simulink model "tx2"  (R2022a)
settings: Solver=FixedStepDiscrete  StartTime=0.0  StopTime=3.1e6  FixedStep=1  RelTol=1e-3
undefined symbols (not defined in the file or in its folder): rom_bf1, rom_bf2, rom_bf3, rom_bf4, rom_bf5, rom_bf6, rom_bf7, rom_bf8, rom_pilot_tt
libraries: hdlsllib x809, whdlutilities x460, whdlmod x104, whdledac x26, simulink x3
(part 20 of 27)

== system tx2/Subsystem7/OFDM_process1/OFDM_process1_bf1/OFDM_BF1 ==
  data : Inport  OutDataTypeStr=fixdt(1,16,14)  LockScale=on
      settings: SignalType=complex
  OFDM_ctrl : Inport  Port=2  OutDataTypeStr=Bus: samplecontrol
  Constant : Constant  Value=0  OutDataTypeStr=boolean
  Data Type Conversion : DataTypeConversion  OutDataTypeStr=boolean  SaturateOnIntegerOverflow=off  RndMeth=Floor
  Delay : Delay  DelayLength=1  InitialCondition=0
  HDL Counter : hdlsllib/Sources/HDL Counter  CountType=Count limited  CountInit=0  CountStep=1  CountMax=1  CountFromType=Initial value  CountFrom=0  CountResetPort=on  CountLoadPort=off  CountEnbPort=on  CountDirPort=off  CountHitOutputPort=off  CountDataType=Unsigned  CountWordLen=8  CountFracLen=0  CountSampTime=1
  HDL Counter1 : hdlsllib/Sources/HDL Counter  CountType=Count limited  CountInit=1  CountStep=1  CountMax=232+cp-1  CountFromType=Initial value  CountFrom=1  CountResetPort=on  CountLoadPort=off  CountEnbPort=on  CountDirPort=off  CountHitOutputPort=on  CountDataType=Unsigned  CountWordLen=10  CountFracLen=0  CountSampTime=1
  Logical Operator1 : Logic  Operator=NOT  AllPortsSameDT=off  OutDataTypeStr=boolean
  OFDM Modulator long prefix : whdlmod/OFDM Modulator  OFDMParametersSource=Property  FFTLength=1024  MaxFFTLength=64  CPLength=cp  numLgSc=0  numRgSc=0  InsertDCNull=off  Windowing=off  WindowLength=cp  MaxWindowLength=8  ResetInputPort=on  Normalize=on  RoundingMethod=Floor  SimulateUsing=Code generation
      settings: SourceProductBaseCode=LH
  Sample Control Bus Selector : whdlutilities/Sample Control Bus Selector  OutputSignals=start,end,valid
      settings: SourceProductBaseCode=LH
  recover_valid_specify : Subsystem  AncestorBlock=mylib/rate_match_L2/interleave/recover_valid_specify
  data_out : Outport  VectorParamsAs1DForOutWhenUnconnected=off
  valid_out : Outport  Port=2  VectorParamsAs1DForOutWhenUnconnected=off
  wires:
  OFDM Modulator long prefix/1 -> data_out/1
  data/1 -> recover_valid_specify/1(data_in)
  OFDM Modulator long prefix/2 -> valid_out/1
  OFDM_ctrl/1 -> Sample Control Bus Selector/1
  Sample Control Bus Selector/2 -> HDL Counter/2  "<end>"
  HDL Counter/1 -> Data Type Conversion/1
  Data Type Conversion/1 -> Logical Operator1/1, HDL Counter1/2
  HDL Counter1/2 -> Delay/1, HDL Counter/1
  Logical Operator1/1 -> HDL Counter1/1
  Sample Control Bus Selector/1 -> recover_valid_specify/2(start_in)  "<start>"
  Delay/1 -> recover_valid_specify/3(end_in)
  recover_valid_specify/1(data_out) -> OFDM Modulator long prefix/1
  recover_valid_specify/4(valid_out) -> OFDM Modulator long prefix/2
  Constant/1 -> OFDM Modulator long prefix/3

== system tx2/Subsystem7/OFDM_process1/OFDM_process1_bf1/ctrl_gen ==
  data_in : Inport
      settings: SignalType=complex
  valid_in : Inport  Port=2
  Delay : Delay  DelayLength=1  InitialCondition=0
  Delay1 : Delay  DelayLength=1  InitialCondition=0
  Delay2 : Delay  DelayLength=1  InitialCondition=0
  Detect Fall Nonpositive : hdlsllib/Logic and Bit Operations/Detect Fall Nonpositive  vinit=0  OutDataTypeStr=boolean
      settings: SourceProductBaseCode=SL
  Detect Rise Positive : hdlsllib/Logic and Bit Operations/Detect Rise Positive  vinit=0  OutDataTypeStr=boolean
      settings: SourceProductBaseCode=SL
  Sample Control Bus Creator : whdlutilities/Sample Control Bus Creator
      settings: SourceProductBaseCode=LH
  data_out : Outport
  ctrl_out : Outport  Port=2
  wires:
  Delay2/1 -> data_out/1
  data_in/1 -> Delay2/1
  Delay1/1 -> Detect Rise Positive/1
  Delay/1 -> Sample Control Bus Creator/3
  Sample Control Bus Creator/1 -> ctrl_out/1
  valid_in/1 -> Delay1/1, Detect Fall Nonpositive/1, Delay/1
  Detect Rise Positive/1 -> Sample Control Bus Creator/1
  Detect Fall Nonpositive/1 -> Sample Control Bus Creator/2

== system tx2/Subsystem7/OFDM_process1/OFDM_process1_bf2/OFDM_BF1 ==
  data : Inport  OutDataTypeStr=fixdt(1,16,14)  LockScale=on
      settings: SignalType=complex
  OFDM_ctrl : Inport  Port=2  OutDataTypeStr=Bus: samplecontrol
  Constant : Constant  Value=0  OutDataTypeStr=boolean
  Data Type Conversion : DataTypeConversion  OutDataTypeStr=boolean  SaturateOnIntegerOverflow=off  RndMeth=Floor
  Delay : Delay  DelayLength=1  InitialCondition=0
  HDL Counter : hdlsllib/Sources/HDL Counter  CountType=Count limited  CountInit=0  CountStep=1  CountMax=1  CountFromType=Initial value  CountFrom=0  CountResetPort=on  CountLoadPort=off  CountEnbPort=on  CountDirPort=off  CountHitOutputPort=off  CountDataType=Unsigned  CountWordLen=8  CountFracLen=0  CountSampTime=1
  HDL Counter1 : hdlsllib/Sources/HDL Counter  CountType=Count limited  CountInit=1  CountStep=1  CountMax=232+cp-1  CountFromType=Initial value  CountFrom=1  CountResetPort=on  CountLoadPort=off  CountEnbPort=on  CountDirPort=off  CountHitOutputPort=on  CountDataType=Unsigned  CountWordLen=10  CountFracLen=0  CountSampTime=1
  Logical Operator1 : Logic  Operator=NOT  AllPortsSameDT=off  OutDataTypeStr=boolean
  OFDM Modulator long prefix : whdlmod/OFDM Modulator  OFDMParametersSource=Property  FFTLength=1024  MaxFFTLength=64  CPLength=cp  numLgSc=0  numRgSc=0  InsertDCNull=off  Windowing=off  WindowLength=cp  MaxWindowLength=8  ResetInputPort=on  Normalize=on  RoundingMethod=Floor  SimulateUsing=Code generation
      settings: SourceProductBaseCode=LH
  Sample Control Bus Selector : whdlutilities/Sample Control Bus Selector  OutputSignals=start,end,valid
      settings: SourceProductBaseCode=LH
  recover_valid_specify : Subsystem  AncestorBlock=mylib/rate_match_L2/interleave/recover_valid_specify
  data_out : Outport  VectorParamsAs1DForOutWhenUnconnected=off
  valid_out : Outport  Port=2  VectorParamsAs1DForOutWhenUnconnected=off
  wires:
  Constant/1 -> OFDM Modulator long prefix/3
  recover_valid_specify/4(valid_out) -> OFDM Modulator long prefix/2
  recover_valid_specify/1(data_out) -> OFDM Modulator long prefix/1
  Delay/1 -> recover_valid_specify/3(end_in)
  Sample Control Bus Selector/1 -> recover_valid_specify/2(start_in)  "<start>"
  Logical Operator1/1 -> HDL Counter1/1
  HDL Counter1/2 -> HDL Counter/1, Delay/1
  Data Type Conversion/1 -> HDL Counter1/2, Logical Operator1/1
  HDL Counter/1 -> Data Type Conversion/1
  Sample Control Bus Selector/2 -> HDL Counter/2  "<end>"
  OFDM_ctrl/1 -> Sample Control Bus Selector/1
  OFDM Modulator long prefix/2 -> valid_out/1
  data/1 -> recover_valid_specify/1(data_in)
  OFDM Modulator long prefix/1 -> data_out/1

== system tx2/Subsystem7/OFDM_process1/OFDM_process1_bf2/ctrl_gen ==
  data_in : Inport
      settings: SignalType=complex
  valid_in : Inport  Port=2
  Delay : Delay  DelayLength=1  InitialCondition=0
  Delay1 : Delay  DelayLength=1  InitialCondition=0
  Delay2 : Delay  DelayLength=1  InitialCondition=0
  Detect Fall Nonpositive : hdlsllib/Logic and Bit Operations/Detect Fall Nonpositive  vinit=0  OutDataTypeStr=boolean
      settings: SourceProductBaseCode=SL
  Detect Rise Positive : hdlsllib/Logic and Bit Operations/Detect Rise Positive  vinit=0  OutDataTypeStr=boolean
      settings: SourceProductBaseCode=SL
  Sample Control Bus Creator : whdlutilities/Sample Control Bus Creator
      settings: SourceProductBaseCode=LH
  data_out : Outport
  ctrl_out : Outport  Port=2
  wires:
  Detect Fall Nonpositive/1 -> Sample Control Bus Creator/2
  Detect Rise Positive/1 -> Sample Control Bus Creator/1
  valid_in/1 -> Delay/1, Detect Fall Nonpositive/1, Delay1/1
  Sample Control Bus Creator/1 -> ctrl_out/1
  Delay/1 -> Sample Control Bus Creator/3
  Delay1/1 -> Detect Rise Positive/1
  data_in/1 -> Delay2/1
  Delay2/1 -> data_out/1

== system tx2/Subsystem7/OFDM_process1/OFDM_process1_bf3/OFDM_BF1 ==
  data : Inport  OutDataTypeStr=fixdt(1,16,14)  LockScale=on
      settings: SignalType=complex
  OFDM_ctrl : Inport  Port=2  OutDataTypeStr=Bus: samplecontrol
  Constant : Constant  Value=0  OutDataTypeStr=boolean
  Data Type Conversion : DataTypeConversion  OutDataTypeStr=boolean  SaturateOnIntegerOverflow=off  RndMeth=Floor
  Delay : Delay  DelayLength=1  InitialCondition=0
  HDL Counter : hdlsllib/Sources/HDL Counter  CountType=Count limited  CountInit=0  CountStep=1  CountMax=1  CountFromType=Initial value  CountFrom=0  CountResetPort=on  CountLoadPort=off  CountEnbPort=on  CountDirPort=off  CountHitOutputPort=off  CountDataType=Unsigned  CountWordLen=8  CountFracLen=0  CountSampTime=1
  HDL Counter1 : hdlsllib/Sources/HDL Counter  CountType=Count limited  CountInit=1  CountStep=1  CountMax=232+cp-1  CountFromType=Initial value  CountFrom=1  CountResetPort=on  CountLoadPort=off  CountEnbPort=on  CountDirPort=off  CountHitOutputPort=on  CountDataType=Unsigned  CountWordLen=10  CountFracLen=0  CountSampTime=1
  Logical Operator1 : Logic  Operator=NOT  AllPortsSameDT=off  OutDataTypeStr=boolean
  OFDM Modulator long prefix : whdlmod/OFDM Modulator  OFDMParametersSource=Property  FFTLength=1024  MaxFFTLength=64  CPLength=cp  numLgSc=0  numRgSc=0  InsertDCNull=off  Windowing=off  WindowLength=cp  MaxWindowLength=8  ResetInputPort=on  Normalize=on  RoundingMethod=Floor  SimulateUsing=Code generation
      settings: SourceProductBaseCode=LH
  Sample Control Bus Selector : whdlutilities/Sample Control Bus Selector  OutputSignals=start,end,valid
      settings: SourceProductBaseCode=LH
  recover_valid_specify : Subsystem  AncestorBlock=mylib/rate_match_L2/interleave/recover_valid_specify
  data_out : Outport  VectorParamsAs1DForOutWhenUnconnected=off
  valid_out : Outport  Port=2  VectorParamsAs1DForOutWhenUnconnected=off
  wires:
  OFDM Modulator long prefix/1 -> data_out/1
  data/1 -> recover_valid_specify/1(data_in)
  OFDM Modulator long prefix/2 -> valid_out/1
  OFDM_ctrl/1 -> Sample Control Bus Selector/1
  Sample Control Bus Selector/2 -> HDL Counter/2  "<end>"
  HDL Counter/1 -> Data Type Conversion/1
  Data Type Conversion/1 -> Logical Operator1/1, HDL Counter1/2
  HDL Counter1/2 -> Delay/1, HDL Counter/1
  Logical Operator1/1 -> HDL Counter1/1
  Sample Control Bus Selector/1 -> recover_valid_specify/2(start_in)  "<start>"
  Delay/1 -> recover_valid_specify/3(end_in)
  recover_valid_specify/1(data_out) -> OFDM Modulator long prefix/1
  recover_valid_specify/4(valid_out) -> OFDM Modulator long prefix/2
  Constant/1 -> OFDM Modulator long prefix/3

== system tx2/Subsystem7/OFDM_process1/OFDM_process1_bf3/ctrl_gen ==
  data_in : Inport
      settings: SignalType=complex
  valid_in : Inport  Port=2
  Delay : Delay  DelayLength=1  InitialCondition=0
  Delay1 : Delay  DelayLength=1  InitialCondition=0
  Delay2 : Delay  DelayLength=1  InitialCondition=0
  Detect Fall Nonpositive : hdlsllib/Logic and Bit Operations/Detect Fall Nonpositive  vinit=0  OutDataTypeStr=boolean
      settings: SourceProductBaseCode=SL
  Detect Rise Positive : hdlsllib/Logic and Bit Operations/Detect Rise Positive  vinit=0  OutDataTypeStr=boolean
      settings: SourceProductBaseCode=SL
  Sample Control Bus Creator : whdlutilities/Sample Control Bus Creator
      settings: SourceProductBaseCode=LH
  data_out : Outport
  ctrl_out : Outport  Port=2
  wires:
  Delay2/1 -> data_out/1
  data_in/1 -> Delay2/1
  Delay1/1 -> Detect Rise Positive/1
  Delay/1 -> Sample Control Bus Creator/3
  Sample Control Bus Creator/1 -> ctrl_out/1
  valid_in/1 -> Delay1/1, Detect Fall Nonpositive/1, Delay/1
  Detect Rise Positive/1 -> Sample Control Bus Creator/1
  Detect Fall Nonpositive/1 -> Sample Control Bus Creator/2

== system tx2/Subsystem7/OFDM_process1/OFDM_process1_bf4/OFDM_BF1 ==
  data : Inport  OutDataTypeStr=fixdt(1,16,14)  LockScale=on
      settings: SignalType=complex
  OFDM_ctrl : Inport  Port=2  OutDataTypeStr=Bus: samplecontrol
  Constant : Constant  Value=0  OutDataTypeStr=boolean
  Data Type Conversion : DataTypeConversion  OutDataTypeStr=boolean  SaturateOnIntegerOverflow=off  RndMeth=Floor
  Delay : Delay  DelayLength=1  InitialCondition=0
  HDL Counter : hdlsllib/Sources/HDL Counter  CountType=Count limited  CountInit=0  CountStep=1  CountMax=1  CountFromType=Initial value  CountFrom=0  CountResetPort=on  CountLoadPort=off  CountEnbPort=on  CountDirPort=off  CountHitOutputPort=off  CountDataType=Unsigned  CountWordLen=8  CountFracLen=0  CountSampTime=1
  HDL Counter1 : hdlsllib/Sources/HDL Counter  CountType=Count limited  CountInit=1  CountStep=1  CountMax=232+cp-1  CountFromType=Initial value  CountFrom=1  CountResetPort=on  CountLoadPort=off  CountEnbPort=on  CountDirPort=off  CountHitOutputPort=on  CountDataType=Unsigned  CountWordLen=10  CountFracLen=0  CountSampTime=1
  Logical Operator1 : Logic  Operator=NOT  AllPortsSameDT=off  OutDataTypeStr=boolean
  OFDM Modulator long prefix : whdlmod/OFDM Modulator  OFDMParametersSource=Property  FFTLength=1024  MaxFFTLength=64  CPLength=cp  numLgSc=0  numRgSc=0  InsertDCNull=off  Windowing=off  WindowLength=cp  MaxWindowLength=8  ResetInputPort=on  Normalize=on  RoundingMethod=Floor  SimulateUsing=Code generation
      settings: SourceProductBaseCode=LH
  Sample Control Bus Selector : whdlutilities/Sample Control Bus Selector  OutputSignals=start,end,valid
      settings: SourceProductBaseCode=LH
  recover_valid_specify : Subsystem  AncestorBlock=mylib/rate_match_L2/interleave/recover_valid_specify
  data_out : Outport  VectorParamsAs1DForOutWhenUnconnected=off
  valid_out : Outport  Port=2  VectorParamsAs1DForOutWhenUnconnected=off
  wires:
  Constant/1 -> OFDM Modulator long prefix/3
  recover_valid_specify/4(valid_out) -> OFDM Modulator long prefix/2
  recover_valid_specify/1(data_out) -> OFDM Modulator long prefix/1
  Delay/1 -> recover_valid_specify/3(end_in)
  Sample Control Bus Selector/1 -> recover_valid_specify/2(start_in)  "<start>"
  Logical Operator1/1 -> HDL Counter1/1
  HDL Counter1/2 -> HDL Counter/1, Delay/1
  Data Type Conversion/1 -> HDL Counter1/2, Logical Operator1/1
  HDL Counter/1 -> Data Type Conversion/1
  Sample Control Bus Selector/2 -> HDL Counter/2  "<end>"
  OFDM_ctrl/1 -> Sample Control Bus Selector/1
  OFDM Modulator long prefix/2 -> valid_out/1
  data/1 -> recover_valid_specify/1(data_in)
  OFDM Modulator long prefix/1 -> data_out/1

== system tx2/Subsystem7/OFDM_process1/OFDM_process1_bf4/ctrl_gen ==
  data_in : Inport
      settings: SignalType=complex
  valid_in : Inport  Port=2
  Delay : Delay  DelayLength=1  InitialCondition=0
  Delay1 : Delay  DelayLength=1  InitialCondition=0
  Delay2 : Delay  DelayLength=1  InitialCondition=0
  Detect Fall Nonpositive : hdlsllib/Logic and Bit Operations/Detect Fall Nonpositive  vinit=0  OutDataTypeStr=boolean
      settings: SourceProductBaseCode=SL
  Detect Rise Positive : hdlsllib/Logic and Bit Operations/Detect Rise Positive  vinit=0  OutDataTypeStr=boolean
      settings: SourceProductBaseCode=SL
  Sample Control Bus Creator : whdlutilities/Sample Control Bus Creator
      settings: SourceProductBaseCode=LH
  data_out : Outport
  ctrl_out : Outport  Port=2
  wires:
  Detect Fall Nonpositive/1 -> Sample Control Bus Creator/2
  Detect Rise Positive/1 -> Sample Control Bus Creator/1
  valid_in/1 -> Delay/1, Detect Fall Nonpositive/1, Delay1/1
  Sample Control Bus Creator/1 -> ctrl_out/1
  Delay/1 -> Sample Control Bus Creator/3
  Delay1/1 -> Detect Rise Positive/1
  data_in/1 -> Delay2/1
  Delay2/1 -> data_out/1

== system tx2/Subsystem7/OFDM_process1/OFDM_process1_bf5/OFDM_BF1 ==
  data : Inport  OutDataTypeStr=fixdt(1,16,14)  LockScale=on
      settings: SignalType=complex
  OFDM_ctrl : Inport  Port=2  OutDataTypeStr=Bus: samplecontrol
  Constant : Constant  Value=0  OutDataTypeStr=boolean
  Data Type Conversion : DataTypeConversion  OutDataTypeStr=boolean  SaturateOnIntegerOverflow=off  RndMeth=Floor
  Delay : Delay  DelayLength=1  InitialCondition=0
  HDL Counter : hdlsllib/Sources/HDL Counter  CountType=Count limited  CountInit=0  CountStep=1  CountMax=1  CountFromType=Initial value  CountFrom=0  CountResetPort=on  CountLoadPort=off  CountEnbPort=on  CountDirPort=off  CountHitOutputPort=off  CountDataType=Unsigned  CountWordLen=8  CountFracLen=0  CountSampTime=1
  HDL Counter1 : hdlsllib/Sources/HDL Counter  CountType=Count limited  CountInit=1  CountStep=1  CountMax=232+cp-1  CountFromType=Initial value  CountFrom=1  CountResetPort=on  CountLoadPort=off  CountEnbPort=on  CountDirPort=off  CountHitOutputPort=on  CountDataType=Unsigned  CountWordLen=10  CountFracLen=0  CountSampTime=1
  Logical Operator1 : Logic  Operator=NOT  AllPortsSameDT=off  OutDataTypeStr=boolean
  OFDM Modulator long prefix : whdlmod/OFDM Modulator  OFDMParametersSource=Property  FFTLength=1024  MaxFFTLength=64  CPLength=cp  numLgSc=0  numRgSc=0  InsertDCNull=off  Windowing=off  WindowLength=cp  MaxWindowLength=8  ResetInputPort=on  Normalize=on  RoundingMethod=Floor  SimulateUsing=Code generation
      settings: SourceProductBaseCode=LH
  Sample Control Bus Selector : whdlutilities/Sample Control Bus Selector  OutputSignals=start,end,valid
      settings: SourceProductBaseCode=LH
  recover_valid_specify : Subsystem  AncestorBlock=mylib/rate_match_L2/interleave/recover_valid_specify
  data_out : Outport  VectorParamsAs1DForOutWhenUnconnected=off
  valid_out : Outport  Port=2  VectorParamsAs1DForOutWhenUnconnected=off
  wires:
  OFDM Modulator long prefix/1 -> data_out/1
  data/1 -> recover_valid_specify/1(data_in)
  OFDM Modulator long prefix/2 -> valid_out/1
  OFDM_ctrl/1 -> Sample Control Bus Selector/1
  Sample Control Bus Selector/2 -> HDL Counter/2  "<end>"
  HDL Counter/1 -> Data Type Conversion/1
  Data Type Conversion/1 -> Logical Operator1/1, HDL Counter1/2
  HDL Counter1/2 -> Delay/1, HDL Counter/1
  Logical Operator1/1 -> HDL Counter1/1
  Sample Control Bus Selector/1 -> recover_valid_specify/2(start_in)  "<start>"
  Delay/1 -> recover_valid_specify/3(end_in)
  recover_valid_specify/1(data_out) -> OFDM Modulator long prefix/1
  recover_valid_specify/4(valid_out) -> OFDM Modulator long prefix/2
  Constant/1 -> OFDM Modulator long prefix/3

== system tx2/Subsystem7/OFDM_process1/OFDM_process1_bf5/ctrl_gen ==
  data_in : Inport
      settings: SignalType=complex
  valid_in : Inport  Port=2
  Delay : Delay  DelayLength=1  InitialCondition=0
  Delay1 : Delay  DelayLength=1  InitialCondition=0
  Delay2 : Delay  DelayLength=1  InitialCondition=0
  Detect Fall Nonpositive : hdlsllib/Logic and Bit Operations/Detect Fall Nonpositive  vinit=0  OutDataTypeStr=boolean
      settings: SourceProductBaseCode=SL
  Detect Rise Positive : hdlsllib/Logic and Bit Operations/Detect Rise Positive  vinit=0  OutDataTypeStr=boolean
      settings: SourceProductBaseCode=SL
  Sample Control Bus Creator : whdlutilities/Sample Control Bus Creator
      settings: SourceProductBaseCode=LH
  data_out : Outport
  ctrl_out : Outport  Port=2
  wires:
  Delay2/1 -> data_out/1
  data_in/1 -> Delay2/1
  Delay1/1 -> Detect Rise Positive/1
  Delay/1 -> Sample Control Bus Creator/3
  Sample Control Bus Creator/1 -> ctrl_out/1
  valid_in/1 -> Delay1/1, Detect Fall Nonpositive/1, Delay/1
  Detect Rise Positive/1 -> Sample Control Bus Creator/1
  Detect Fall Nonpositive/1 -> Sample Control Bus Creator/2

== system tx2/Subsystem7/OFDM_process1/OFDM_process1_bf6/OFDM_BF1 ==
  data : Inport  OutDataTypeStr=fixdt(1,16,14)  LockScale=on
      settings: SignalType=complex
  OFDM_ctrl : Inport  Port=2  OutDataTypeStr=Bus: samplecontrol
  Constant : Constant  Value=0  OutDataTypeStr=boolean
  Data Type Conversion : DataTypeConversion  OutDataTypeStr=boolean  SaturateOnIntegerOverflow=off  RndMeth=Floor
  Delay : Delay  DelayLength=1  InitialCondition=0
  HDL Counter : hdlsllib/Sources/HDL Counter  CountType=Count limited  CountInit=0  CountStep=1  CountMax=1  CountFromType=Initial value  CountFrom=0  CountResetPort=on  CountLoadPort=off  CountEnbPort=on  CountDirPort=off  CountHitOutputPort=off  CountDataType=Unsigned  CountWordLen=8  CountFracLen=0  CountSampTime=1
  HDL Counter1 : hdlsllib/Sources/HDL Counter  CountType=Count limited  CountInit=1  CountStep=1  CountMax=232+cp-1  CountFromType=Initial value  CountFrom=1  CountResetPort=on  CountLoadPort=off  CountEnbPort=on  CountDirPort=off  CountHitOutputPort=on  CountDataType=Unsigned  CountWordLen=10  CountFracLen=0  CountSampTime=1
  Logical Operator1 : Logic  Operator=NOT  AllPortsSameDT=off  OutDataTypeStr=boolean
  OFDM Modulator long prefix : whdlmod/OFDM Modulator  OFDMParametersSource=Property  FFTLength=1024  MaxFFTLength=64  CPLength=cp  numLgSc=0  numRgSc=0  InsertDCNull=off  Windowing=off  WindowLength=cp  MaxWindowLength=8  ResetInputPort=on  Normalize=on  RoundingMethod=Floor  SimulateUsing=Code generation
      settings: SourceProductBaseCode=LH
  Sample Control Bus Selector : whdlutilities/Sample Control Bus Selector  OutputSignals=start,end,valid
      settings: SourceProductBaseCode=LH
  recover_valid_specify : Subsystem  AncestorBlock=mylib/rate_match_L2/interleave/recover_valid_specify
  data_out : Outport  VectorParamsAs1DForOutWhenUnconnected=off
  valid_out : Outport  Port=2  VectorParamsAs1DForOutWhenUnconnected=off
  wires:
  Constant/1 -> OFDM Modulator long prefix/3
  recover_valid_specify/4(valid_out) -> OFDM Modulator long prefix/2
  recover_valid_specify/1(data_out) -> OFDM Modulator long prefix/1
  Delay/1 -> recover_valid_specify/3(end_in)
  Sample Control Bus Selector/1 -> recover_valid_specify/2(start_in)  "<start>"
  Logical Operator1/1 -> HDL Counter1/1
  HDL Counter1/2 -> HDL Counter/1, Delay/1
  Data Type Conversion/1 -> HDL Counter1/2, Logical Operator1/1
  HDL Counter/1 -> Data Type Conversion/1
  Sample Control Bus Selector/2 -> HDL Counter/2  "<end>"
  OFDM_ctrl/1 -> Sample Control Bus Selector/1
  OFDM Modulator long prefix/2 -> valid_out/1
  data/1 -> recover_valid_specify/1(data_in)
  OFDM Modulator long prefix/1 -> data_out/1

== system tx2/Subsystem7/OFDM_process1/OFDM_process1_bf6/ctrl_gen ==
  data_in : Inport
      settings: SignalType=complex
  valid_in : Inport  Port=2
  Delay : Delay  DelayLength=1  InitialCondition=0
  Delay1 : Delay  DelayLength=1  InitialCondition=0
  Delay2 : Delay  DelayLength=1  InitialCondition=0
  Detect Fall Nonpositive : hdlsllib/Logic and Bit Operations/Detect Fall Nonpositive  vinit=0  OutDataTypeStr=boolean
      settings: SourceProductBaseCode=SL
  Detect Rise Positive : hdlsllib/Logic and Bit Operations/Detect Rise Positive  vinit=0  OutDataTypeStr=boolean
      settings: SourceProductBaseCode=SL
  Sample Control Bus Creator : whdlutilities/Sample Control Bus Creator
      settings: SourceProductBaseCode=LH
  data_out : Outport
  ctrl_out : Outport  Port=2
  wires:
  Detect Fall Nonpositive/1 -> Sample Control Bus Creator/2
  Detect Rise Positive/1 -> Sample Control Bus Creator/1
  valid_in/1 -> Delay/1, Detect Fall Nonpositive/1, Delay1/1
  Sample Control Bus Creator/1 -> ctrl_out/1
  Delay/1 -> Sample Control Bus Creator/3
  Delay1/1 -> Detect Rise Positive/1
  data_in/1 -> Delay2/1
  Delay2/1 -> data_out/1

== system tx2/Subsystem7/OFDM_process1/OFDM_process1_bf7/OFDM_BF1 ==
  data : Inport  OutDataTypeStr=fixdt(1,16,14)  LockScale=on
      settings: SignalType=complex
  OFDM_ctrl : Inport  Port=2  OutDataTypeStr=Bus: samplecontrol
  Constant : Constant  Value=0  OutDataTypeStr=boolean
  Data Type Conversion : DataTypeConversion  OutDataTypeStr=boolean  SaturateOnIntegerOverflow=off  RndMeth=Floor
  Delay : Delay  DelayLength=1  InitialCondition=0
  HDL Counter : hdlsllib/Sources/HDL Counter  CountType=Count limited  CountInit=0  CountStep=1  CountMax=1  CountFromType=Initial value  CountFrom=0  CountResetPort=on  CountLoadPort=off  CountEnbPort=on  CountDirPort=off  CountHitOutputPort=off  CountDataType=Unsigned  CountWordLen=8  CountFracLen=0  CountSampTime=1
  HDL Counter1 : hdlsllib/Sources/HDL Counter  CountType=Count limited  CountInit=1  CountStep=1  CountMax=232+cp-1  CountFromType=Initial value  CountFrom=1  CountResetPort=on  CountLoadPort=off  CountEnbPort=on  CountDirPort=off  CountHitOutputPort=on  CountDataType=Unsigned  CountWordLen=10  CountFracLen=0  CountSampTime=1
  Logical Operator1 : Logic  Operator=NOT  AllPortsSameDT=off  OutDataTypeStr=boolean
  OFDM Modulator long prefix : whdlmod/OFDM Modulator  OFDMParametersSource=Property  FFTLength=1024  MaxFFTLength=64  CPLength=cp  numLgSc=0  numRgSc=0  InsertDCNull=off  Windowing=off  WindowLength=cp  MaxWindowLength=8  ResetInputPort=on  Normalize=on  RoundingMethod=Floor  SimulateUsing=Code generation
      settings: SourceProductBaseCode=LH
  Sample Control Bus Selector : whdlutilities/Sample Control Bus Selector  OutputSignals=start,end,valid
      settings: SourceProductBaseCode=LH
  recover_valid_specify : Subsystem  AncestorBlock=mylib/rate_match_L2/interleave/recover_valid_specify
  data_out : Outport  VectorParamsAs1DForOutWhenUnconnected=off
  valid_out : Outport  Port=2  VectorParamsAs1DForOutWhenUnconnected=off
  wires:
  OFDM Modulator long prefix/1 -> data_out/1
  data/1 -> recover_valid_specify/1(data_in)
  OFDM Modulator long prefix/2 -> valid_out/1
  OFDM_ctrl/1 -> Sample Control Bus Selector/1
  Sample Control Bus Selector/2 -> HDL Counter/2  "<end>"
  HDL Counter/1 -> Data Type Conversion/1
  Data Type Conversion/1 -> Logical Operator1/1, HDL Counter1/2
  HDL Counter1/2 -> Delay/1, HDL Counter/1
  Logical Operator1/1 -> HDL Counter1/1
  Sample Control Bus Selector/1 -> recover_valid_specify/2(start_in)  "<start>"
  Delay/1 -> recover_valid_specify/3(end_in)
  recover_valid_specify/1(data_out) -> OFDM Modulator long prefix/1
  recover_valid_specify/4(valid_out) -> OFDM Modulator long prefix/2
  Constant/1 -> OFDM Modulator long prefix/3

== system tx2/Subsystem7/OFDM_process1/OFDM_process1_bf7/ctrl_gen ==
  data_in : Inport
      settings: SignalType=complex
  valid_in : Inport  Port=2
  Delay : Delay  DelayLength=1  InitialCondition=0
  Delay1 : Delay  DelayLength=1  InitialCondition=0
  Delay2 : Delay  DelayLength=1  InitialCondition=0
  Detect Fall Nonpositive : hdlsllib/Logic and Bit Operations/Detect Fall Nonpositive  vinit=0  OutDataTypeStr=boolean
      settings: SourceProductBaseCode=SL
  Detect Rise Positive : hdlsllib/Logic and Bit Operations/Detect Rise Positive  vinit=0  OutDataTypeStr=boolean
      settings: SourceProductBaseCode=SL
  Sample Control Bus Creator : whdlutilities/Sample Control Bus Creator
      settings: SourceProductBaseCode=LH
  data_out : Outport
  ctrl_out : Outport  Port=2
  wires:
  Delay2/1 -> data_out/1
  data_in/1 -> Delay2/1
  Delay1/1 -> Detect Rise Positive/1
  Delay/1 -> Sample Control Bus Creator/3
  Sample Control Bus Creator/1 -> ctrl_out/1
  valid_in/1 -> Delay1/1, Detect Fall Nonpositive/1, Delay/1
  Detect Rise Positive/1 -> Sample Control Bus Creator/1
  Detect Fall Nonpositive/1 -> Sample Control Bus Creator/2

== system tx2/Subsystem7/OFDM_process1/OFDM_process1_bf8/OFDM_BF1 ==
  data : Inport  OutDataTypeStr=fixdt(1,16,14)  LockScale=on
      settings: SignalType=complex
  OFDM_ctrl : Inport  Port=2  OutDataTypeStr=Bus: samplecontrol
  Constant : Constant  Value=0  OutDataTypeStr=boolean
  Data Type Conversion : DataTypeConversion  OutDataTypeStr=boolean  SaturateOnIntegerOverflow=off  RndMeth=Floor
  Delay : Delay  DelayLength=1  InitialCondition=0
  HDL Counter : hdlsllib/Sources/HDL Counter  CountType=Count limited  CountInit=0  CountStep=1  CountMax=1  CountFromType=Initial value  CountFrom=0  CountResetPort=on  CountLoadPort=off  CountEnbPort=on  CountDirPort=off  CountHitOutputPort=off  CountDataType=Unsigned  CountWordLen=8  CountFracLen=0  CountSampTime=1
  HDL Counter1 : hdlsllib/Sources/HDL Counter  CountType=Count limited  CountInit=1  CountStep=1  CountMax=232+cp-1  CountFromType=Initial value  CountFrom=1  CountResetPort=on  CountLoadPort=off  CountEnbPort=on  CountDirPort=off  CountHitOutputPort=on  CountDataType=Unsigned  CountWordLen=10  CountFracLen=0  CountSampTime=1
  Logical Operator1 : Logic  Operator=NOT  AllPortsSameDT=off  OutDataTypeStr=boolean
  OFDM Modulator long prefix : whdlmod/OFDM Modulator  OFDMParametersSource=Property  FFTLength=1024  MaxFFTLength=64  CPLength=cp  numLgSc=0  numRgSc=0  InsertDCNull=off  Windowing=off  WindowLength=cp  MaxWindowLength=8  ResetInputPort=on  Normalize=on  RoundingMethod=Floor  SimulateUsing=Code generation
      settings: SourceProductBaseCode=LH
  Sample Control Bus Selector : whdlutilities/Sample Control Bus Selector  OutputSignals=start,end,valid
      settings: SourceProductBaseCode=LH
  recover_valid_specify : Subsystem  AncestorBlock=mylib/rate_match_L2/interleave/recover_valid_specify
  data_out : Outport  VectorParamsAs1DForOutWhenUnconnected=off
  valid_out : Outport  Port=2  VectorParamsAs1DForOutWhenUnconnected=off
  wires:
  Constant/1 -> OFDM Modulator long prefix/3
  recover_valid_specify/4(valid_out) -> OFDM Modulator long prefix/2
  recover_valid_specify/1(data_out) -> OFDM Modulator long prefix/1
  Delay/1 -> recover_valid_specify/3(end_in)
  Sample Control Bus Selector/1 -> recover_valid_specify/2(start_in)  "<start>"
  Logical Operator1/1 -> HDL Counter1/1
  HDL Counter1/2 -> HDL Counter/1, Delay/1
  Data Type Conversion/1 -> HDL Counter1/2, Logical Operator1/1
  HDL Counter/1 -> Data Type Conversion/1
  Sample Control Bus Selector/2 -> HDL Counter/2  "<end>"
  OFDM_ctrl/1 -> Sample Control Bus Selector/1
  OFDM Modulator long prefix/2 -> valid_out/1
  data/1 -> recover_valid_specify/1(data_in)
  OFDM Modulator long prefix/1 -> data_out/1

== system tx2/Subsystem7/OFDM_process1/OFDM_process1_bf8/ctrl_gen ==
  data_in : Inport
      settings: SignalType=complex
  valid_in : Inport  Port=2
  Delay : Delay  DelayLength=1  InitialCondition=0
  Delay1 : Delay  DelayLength=1  InitialCondition=0
  Delay2 : Delay  DelayLength=1  InitialCondition=0
  Detect Fall Nonpositive : hdlsllib/Logic and Bit Operations/Detect Fall Nonpositive  vinit=0  OutDataTypeStr=boolean
      settings: SourceProductBaseCode=SL
  Detect Rise Positive : hdlsllib/Logic and Bit Operations/Detect Rise Positive  vinit=0  OutDataTypeStr=boolean
      settings: SourceProductBaseCode=SL
  Sample Control Bus Creator : whdlutilities/Sample Control Bus Creator
      settings: SourceProductBaseCode=LH
  data_out : Outport
  ctrl_out : Outport  Port=2
  wires:
  Detect Fall Nonpositive/1 -> Sample Control Bus Creator/2
  Detect Rise Positive/1 -> Sample Control Bus Creator/1
  valid_in/1 -> Delay/1, Detect Fall Nonpositive/1, Delay1/1
  Sample Control Bus Creator/1 -> ctrl_out/1
  Delay/1 -> Sample Control Bus Creator/3
  Delay1/1 -> Detect Rise Positive/1
  data_in/1 -> Delay2/1
  Delay2/1 -> data_out/1

== system tx2/Subsystem7/bit_level/ctrl_gen/ctrl_gen ==
  data_in : Inport
  valid_in : Inport  Port=2
  Delay : Delay  DelayLength=1  InitialCondition=0
  Delay1 : Delay  DelayLength=1  InitialCondition=0
  Delay2 : Delay  DelayLength=1  InitialCondition=0
  Detect Fall Nonpositive : hdlsllib/Logic and Bit Operations/Detect Fall Nonpositive  vinit=0  OutDataTypeStr=boolean
      settings: SourceProductBaseCode=SL
  Detect Rise Positive : hdlsllib/Logic and Bit Operations/Detect Rise Positive  vinit=0  OutDataTypeStr=boolean
      settings: SourceProductBaseCode=SL
  Sample Control Bus Creator : whdlutilities/Sample Control Bus Creator
      settings: SourceProductBaseCode=LH
  data_out : Outport
  ctrl_out : Outport  Port=2
  wires:
  Detect Fall Nonpositive/1 -> Sample Control Bus Creator/2
  Detect Rise Positive/1 -> Sample Control Bus Creator/1
  valid_in/1 -> Delay/1, Detect Fall Nonpositive/1, Delay1/1
  Sample Control Bus Creator/1 -> ctrl_out/1
  Delay/1 -> Sample Control Bus Creator/3
  Delay1/1 -> Detect Rise Positive/1
  data_in/1 -> Delay2/1
  Delay2/1 -> data_out/1

== system tx2/Subsystem8/BF/rom_bf1/HDL ROM ==
  note: NumAntRRU = 8;
      | beamforming = sqrt(1/NumAntRRU) * exp( -2j*pi*(1-1)/NumAntRRU ...
      | .*(0:NumAntRRU-1) )';
      | beamforming = fi(beamforming,1,16,8)
  rom_address : Inport
  Direct Lookup Table (n-D) : LookupNDDirect  NumberOfTableDimensions=1  Table=rom_bf1  DiagnosticForOutOfRangeInput=Error
  ResetNoneDelay : Delay  DelayLength=1
  data_out : Outport
  wires:
  ResetNoneDelay/1 -> data_out/1
  Direct Lookup Table (n-D)/1 -> ResetNoneDelay/1
  rom_address/1 -> Direct Lookup Table (n-D)/1

== system tx2/Subsystem8/BF/rom_bf2/HDL ROM ==
  note: NumAntRRU = 8;
      | beamforming = sqrt(1/NumAntRRU) * exp( -2j*pi*(1-1)/NumAntRRU ...
      | .*(0:NumAntRRU-1) )';
      | beamforming = fi(beamforming,1,16,8)
  rom_address : Inport
  Direct Lookup Table (n-D) : LookupNDDirect  NumberOfTableDimensions=1  Table=rom_bf2  DiagnosticForOutOfRangeInput=Error
  ResetNoneDelay : Delay  DelayLength=1
  data_out : Outport
  wires:
  rom_address/1 -> Direct Lookup Table (n-D)/1
  Direct Lookup Table (n-D)/1 -> ResetNoneDelay/1
  ResetNoneDelay/1 -> data_out/1

== system tx2/Subsystem8/BF/rom_bf3/HDL ROM ==
  note: NumAntRRU = 8;
      | beamforming = sqrt(1/NumAntRRU) * exp( -2j*pi*(1-1)/NumAntRRU ...
      | .*(0:NumAntRRU-1) )';
      | beamforming = fi(beamforming,1,16,8)
  rom_address : Inport
  Direct Lookup Table (n-D) : LookupNDDirect  NumberOfTableDimensions=1  Table=rom_bf3  DiagnosticForOutOfRangeInput=Error
  ResetNoneDelay : Delay  DelayLength=1
  data_out : Outport
  wires:
  ResetNoneDelay/1 -> data_out/1
  Direct Lookup Table (n-D)/1 -> ResetNoneDelay/1
  rom_address/1 -> Direct Lookup Table (n-D)/1

== system tx2/Subsystem8/BF/rom_bf4/HDL ROM ==
  note: NumAntRRU = 8;
      | beamforming = sqrt(1/NumAntRRU) * exp( -2j*pi*(1-1)/NumAntRRU ...
      | .*(0:NumAntRRU-1) )';
      | beamforming = fi(beamforming,1,16,8)
  rom_address : Inport
  Direct Lookup Table (n-D) : LookupNDDirect  NumberOfTableDimensions=1  Table=rom_bf4  DiagnosticForOutOfRangeInput=Error
  ResetNoneDelay : Delay  DelayLength=1
  data_out : Outport
  wires:
  rom_address/1 -> Direct Lookup Table (n-D)/1
  Direct Lookup Table (n-D)/1 -> ResetNoneDelay/1
  ResetNoneDelay/1 -> data_out/1

== system tx2/Subsystem8/BF/rom_bf5/HDL ROM ==
  note: NumAntRRU = 8;
      | beamforming = sqrt(1/NumAntRRU) * exp( -2j*pi*(1-1)/NumAntRRU ...
      | .*(0:NumAntRRU-1) )';
      | beamforming = fi(beamforming,1,16,8)
  rom_address : Inport
  Direct Lookup Table (n-D) : LookupNDDirect  NumberOfTableDimensions=1  Table=rom_bf5  DiagnosticForOutOfRangeInput=Error
  ResetNoneDelay : Delay  DelayLength=1
  data_out : Outport
  wires:
  ResetNoneDelay/1 -> data_out/1
  Direct Lookup Table (n-D)/1 -> ResetNoneDelay/1
  rom_address/1 -> Direct Lookup Table (n-D)/1

== system tx2/Subsystem8/BF/rom_bf6/HDL ROM ==
  note: NumAntRRU = 8;
      | beamforming = sqrt(1/NumAntRRU) * exp( -2j*pi*(1-1)/NumAntRRU ...
      | .*(0:NumAntRRU-1) )';
      | beamforming = fi(beamforming,1,16,8)
  rom_address : Inport
  Direct Lookup Table (n-D) : LookupNDDirect  NumberOfTableDimensions=1  Table=rom_bf6  DiagnosticForOutOfRangeInput=Error
  ResetNoneDelay : Delay  DelayLength=1
  data_out : Outport
  wires:
  rom_address/1 -> Direct Lookup Table (n-D)/1
  Direct Lookup Table (n-D)/1 -> ResetNoneDelay/1
  ResetNoneDelay/1 -> data_out/1

== system tx2/Subsystem8/BF/rom_bf7/HDL ROM ==
  note: NumAntRRU = 8;
      | beamforming = sqrt(1/NumAntRRU) * exp( -2j*pi*(1-1)/NumAntRRU ...
      | .*(0:NumAntRRU-1) )';
      | beamforming = fi(beamforming,1,16,8)
  rom_address : Inport
  Direct Lookup Table (n-D) : LookupNDDirect  NumberOfTableDimensions=1  Table=rom_bf7  DiagnosticForOutOfRangeInput=Error
  ResetNoneDelay : Delay  DelayLength=1
  data_out : Outport
  wires:
  ResetNoneDelay/1 -> data_out/1
  Direct Lookup Table (n-D)/1 -> ResetNoneDelay/1
  rom_address/1 -> Direct Lookup Table (n-D)/1

== system tx2/Subsystem8/BF/rom_bf8/HDL ROM ==
  note: NumAntRRU = 8;
      | beamforming = sqrt(1/NumAntRRU) * exp( -2j*pi*(1-1)/NumAntRRU ...
      | .*(0:NumAntRRU-1) )';
      | beamforming = fi(beamforming,1,16,8)
  rom_address : Inport
  Direct Lookup Table (n-D) : LookupNDDirect  NumberOfTableDimensions=1  Table=rom_bf8  DiagnosticForOutOfRangeInput=Error
  ResetNoneDelay : Delay  DelayLength=1
  data_out : Outport
  wires:
  rom_address/1 -> Direct Lookup Table (n-D)/1
  Direct Lookup Table (n-D)/1 -> ResetNoneDelay/1
  ResetNoneDelay/1 -> data_out/1

== system tx2/Subsystem8/OFDM_process1/OFDM_process1_bf1/OFDM_BF1 ==
  data : Inport  OutDataTypeStr=fixdt(1,16,14)  LockScale=on
      settings: SignalType=complex
  OFDM_ctrl : Inport  Port=2  OutDataTypeStr=Bus: samplecontrol
  Constant : Constant  Value=0  OutDataTypeStr=boolean
  Data Type Conversion : DataTypeConversion  OutDataTypeStr=boolean  SaturateOnIntegerOverflow=off  RndMeth=Floor
  Delay : Delay  DelayLength=1  InitialCondition=0
  HDL Counter : hdlsllib/Sources/HDL Counter  CountType=Count limited  CountInit=0  CountStep=1  CountMax=1  CountFromType=Initial value  CountFrom=0  CountResetPort=on  CountLoadPort=off  CountEnbPort=on  CountDirPort=off  CountHitOutputPort=off  CountDataType=Unsigned  CountWordLen=8  CountFracLen=0  CountSampTime=1
  HDL Counter1 : hdlsllib/Sources/HDL Counter  CountType=Count limited  CountInit=1  CountStep=1  CountMax=232+cp-1  CountFromType=Initial value  CountFrom=1  CountResetPort=on  CountLoadPort=off  CountEnbPort=on  CountDirPort=off  CountHitOutputPort=on  CountDataType=Unsigned  CountWordLen=10  CountFracLen=0  CountSampTime=1
  Logical Operator1 : Logic  Operator=NOT  AllPortsSameDT=off  OutDataTypeStr=boolean
  OFDM Modulator long prefix : whdlmod/OFDM Modulator  OFDMParametersSource=Property  FFTLength=1024  MaxFFTLength=64  CPLength=cp  numLgSc=0  numRgSc=0  InsertDCNull=off  Windowing=off  WindowLength=cp  MaxWindowLength=8  ResetInputPort=on  Normalize=on  RoundingMethod=Floor  SimulateUsing=Code generation
      settings: SourceProductBaseCode=LH
  Sample Control Bus Selector : whdlutilities/Sample Control Bus Selector  OutputSignals=start,end,valid
      settings: SourceProductBaseCode=LH
  recover_valid_specify : Subsystem  AncestorBlock=mylib/rate_match_L2/interleave/recover_valid_specify
  data_out : Outport  VectorParamsAs1DForOutWhenUnconnected=off
  valid_out : Outport  Port=2  VectorParamsAs1DForOutWhenUnconnected=off
  wires:
  Constant/1 -> OFDM Modulator long prefix/3
  recover_valid_specify/4(valid_out) -> OFDM Modulator long prefix/2
  recover_valid_specify/1(data_out) -> OFDM Modulator long prefix/1
  Delay/1 -> recover_valid_specify/3(end_in)
  Sample Control Bus Selector/1 -> recover_valid_specify/2(start_in)  "<start>"
  Logical Operator1/1 -> HDL Counter1/1
  HDL Counter1/2 -> HDL Counter/1, Delay/1
  Data Type Conversion/1 -> HDL Counter1/2, Logical Operator1/1
  HDL Counter/1 -> Data Type Conversion/1
  Sample Control Bus Selector/2 -> HDL Counter/2  "<end>"
  OFDM_ctrl/1 -> Sample Control Bus Selector/1
  OFDM Modulator long prefix/2 -> valid_out/1
  data/1 -> recover_valid_specify/1(data_in)
  OFDM Modulator long prefix/1 -> data_out/1

== system tx2/Subsystem8/OFDM_process1/OFDM_process1_bf1/ctrl_gen ==
  data_in : Inport
      settings: SignalType=complex
  valid_in : Inport  Port=2
  Delay : Delay  DelayLength=1  InitialCondition=0
  Delay1 : Delay  DelayLength=1  InitialCondition=0
  Delay2 : Delay  DelayLength=1  InitialCondition=0
  Detect Fall Nonpositive : hdlsllib/Logic and Bit Operations/Detect Fall Nonpositive  vinit=0  OutDataTypeStr=boolean
      settings: SourceProductBaseCode=SL
  Detect Rise Positive : hdlsllib/Logic and Bit Operations/Detect Rise Positive  vinit=0  OutDataTypeStr=boolean
      settings: SourceProductBaseCode=SL
  Sample Control Bus Creator : whdlutilities/Sample Control Bus Creator
      settings: SourceProductBaseCode=LH
  data_out : Outport
  ctrl_out : Outport  Port=2
  wires:
  Detect Fall Nonpositive/1 -> Sample Control Bus Creator/2
  Detect Rise Positive/1 -> Sample Control Bus Creator/1
  valid_in/1 -> Delay/1, Detect Fall Nonpositive/1, Delay1/1
  Sample Control Bus Creator/1 -> ctrl_out/1
  Delay/1 -> Sample Control Bus Creator/3
  Delay1/1 -> Detect Rise Positive/1
  data_in/1 -> Delay2/1
  Delay2/1 -> data_out/1

== system tx2/Subsystem8/OFDM_process1/OFDM_process1_bf2/OFDM_BF1 ==
  data : Inport  OutDataTypeStr=fixdt(1,16,14)  LockScale=on
      settings: SignalType=complex
  OFDM_ctrl : Inport  Port=2  OutDataTypeStr=Bus: samplecontrol
  Constant : Constant  Value=0  OutDataTypeStr=boolean
  Data Type Conversion : DataTypeConversion  OutDataTypeStr=boolean  SaturateOnIntegerOverflow=off  RndMeth=Floor
  Delay : Delay  DelayLength=1  InitialCondition=0
  HDL Counter : hdlsllib/Sources/HDL Counter  CountType=Count limited  CountInit=0  CountStep=1  CountMax=1  CountFromType=Initial value  CountFrom=0  CountResetPort=on  CountLoadPort=off  CountEnbPort=on  CountDirPort=off  CountHitOutputPort=off  CountDataType=Unsigned  CountWordLen=8  CountFracLen=0  CountSampTime=1
  HDL Counter1 : hdlsllib/Sources/HDL Counter  CountType=Count limited  CountInit=1  CountStep=1  CountMax=232+cp-1  CountFromType=Initial value  CountFrom=1  CountResetPort=on  CountLoadPort=off  CountEnbPort=on  CountDirPort=off  CountHitOutputPort=on  CountDataType=Unsigned  CountWordLen=10  CountFracLen=0  CountSampTime=1
  Logical Operator1 : Logic  Operator=NOT  AllPortsSameDT=off  OutDataTypeStr=boolean
  OFDM Modulator long prefix : whdlmod/OFDM Modulator  OFDMParametersSource=Property  FFTLength=1024  MaxFFTLength=64  CPLength=cp  numLgSc=0  numRgSc=0  InsertDCNull=off  Windowing=off  WindowLength=cp  MaxWindowLength=8  ResetInputPort=on  Normalize=on  RoundingMethod=Floor  SimulateUsing=Code generation
      settings: SourceProductBaseCode=LH
  Sample Control Bus Selector : whdlutilities/Sample Control Bus Selector  OutputSignals=start,end,valid
      settings: SourceProductBaseCode=LH
  recover_valid_specify : Subsystem  AncestorBlock=mylib/rate_match_L2/interleave/recover_valid_specify
  data_out : Outport  VectorParamsAs1DForOutWhenUnconnected=off
  valid_out : Outport  Port=2  VectorParamsAs1DForOutWhenUnconnected=off
  wires:
  OFDM Modulator long prefix/1 -> data_out/1
  data/1 -> recover_valid_specify/1(data_in)
  OFDM Modulator long prefix/2 -> valid_out/1
  OFDM_ctrl/1 -> Sample Control Bus Selector/1
  Sample Control Bus Selector/2 -> HDL Counter/2  "<end>"
  HDL Counter/1 -> Data Type Conversion/1
  Data Type Conversion/1 -> Logical Operator1/1, HDL Counter1/2
  HDL Counter1/2 -> Delay/1, HDL Counter/1
  Logical Operator1/1 -> HDL Counter1/1
  Sample Control Bus Selector/1 -> recover_valid_specify/2(start_in)  "<start>"
  Delay/1 -> recover_valid_specify/3(end_in)
  recover_valid_specify/1(data_out) -> OFDM Modulator long prefix/1
  recover_valid_specify/4(valid_out) -> OFDM Modulator long prefix/2
  Constant/1 -> OFDM Modulator long prefix/3

== system tx2/Subsystem8/OFDM_process1/OFDM_process1_bf2/ctrl_gen ==
  data_in : Inport
      settings: SignalType=complex
  valid_in : Inport  Port=2
  Delay : Delay  DelayLength=1  InitialCondition=0
  Delay1 : Delay  DelayLength=1  InitialCondition=0
  Delay2 : Delay  DelayLength=1  InitialCondition=0
  Detect Fall Nonpositive : hdlsllib/Logic and Bit Operations/Detect Fall Nonpositive  vinit=0  OutDataTypeStr=boolean
      settings: SourceProductBaseCode=SL
  Detect Rise Positive : hdlsllib/Logic and Bit Operations/Detect Rise Positive  vinit=0  OutDataTypeStr=boolean
      settings: SourceProductBaseCode=SL
  Sample Control Bus Creator : whdlutilities/Sample Control Bus Creator
      settings: SourceProductBaseCode=LH
  data_out : Outport
  ctrl_out : Outport  Port=2
  wires:
  Delay2/1 -> data_out/1
  data_in/1 -> Delay2/1
  Delay1/1 -> Detect Rise Positive/1
  Delay/1 -> Sample Control Bus Creator/3
  Sample Control Bus Creator/1 -> ctrl_out/1
  valid_in/1 -> Delay1/1, Detect Fall Nonpositive/1, Delay/1
  Detect Rise Positive/1 -> Sample Control Bus Creator/1
  Detect Fall Nonpositive/1 -> Sample Control Bus Creator/2

== system tx2/Subsystem8/OFDM_process1/OFDM_process1_bf3/OFDM_BF1 ==
  data : Inport  OutDataTypeStr=fixdt(1,16,14)  LockScale=on
      settings: SignalType=complex
  OFDM_ctrl : Inport  Port=2  OutDataTypeStr=Bus: samplecontrol
  Constant : Constant  Value=0  OutDataTypeStr=boolean
  Data Type Conversion : DataTypeConversion  OutDataTypeStr=boolean  SaturateOnIntegerOverflow=off  RndMeth=Floor
  Delay : Delay  DelayLength=1  InitialCondition=0
  HDL Counter : hdlsllib/Sources/HDL Counter  CountType=Count limited  CountInit=0  CountStep=1  CountMax=1  CountFromType=Initial value  CountFrom=0  CountResetPort=on  CountLoadPort=off  CountEnbPort=on  CountDirPort=off  CountHitOutputPort=off  CountDataType=Unsigned  CountWordLen=8  CountFracLen=0  CountSampTime=1
  HDL Counter1 : hdlsllib/Sources/HDL Counter  CountType=Count limited  CountInit=1  CountStep=1  CountMax=232+cp-1  CountFromType=Initial value  CountFrom=1  CountResetPort=on  CountLoadPort=off  CountEnbPort=on  CountDirPort=off  CountHitOutputPort=on  CountDataType=Unsigned  CountWordLen=10  CountFracLen=0  CountSampTime=1
  Logical Operator1 : Logic  Operator=NOT  AllPortsSameDT=off  OutDataTypeStr=boolean
  OFDM Modulator long prefix : whdlmod/OFDM Modulator  OFDMParametersSource=Property  FFTLength=1024  MaxFFTLength=64  CPLength=cp  numLgSc=0  numRgSc=0  InsertDCNull=off  Windowing=off  WindowLength=cp  MaxWindowLength=8  ResetInputPort=on  Normalize=on  RoundingMethod=Floor  SimulateUsing=Code generation
      settings: SourceProductBaseCode=LH
  Sample Control Bus Selector : whdlutilities/Sample Control Bus Selector  OutputSignals=start,end,valid
      settings: SourceProductBaseCode=LH
  recover_valid_specify : Subsystem  AncestorBlock=mylib/rate_match_L2/interleave/recover_valid_specify
  data_out : Outport  VectorParamsAs1DForOutWhenUnconnected=off
  valid_out : Outport  Port=2  VectorParamsAs1DForOutWhenUnconnected=off
  wires:
  Constant/1 -> OFDM Modulator long prefix/3
  recover_valid_specify/4(valid_out) -> OFDM Modulator long prefix/2
  recover_valid_specify/1(data_out) -> OFDM Modulator long prefix/1
  Delay/1 -> recover_valid_specify/3(end_in)
  Sample Control Bus Selector/1 -> recover_valid_specify/2(start_in)  "<start>"
  Logical Operator1/1 -> HDL Counter1/1
  HDL Counter1/2 -> HDL Counter/1, Delay/1
  Data Type Conversion/1 -> HDL Counter1/2, Logical Operator1/1
  HDL Counter/1 -> Data Type Conversion/1
  Sample Control Bus Selector/2 -> HDL Counter/2  "<end>"
  OFDM_ctrl/1 -> Sample Control Bus Selector/1
  OFDM Modulator long prefix/2 -> valid_out/1
  data/1 -> recover_valid_specify/1(data_in)
  OFDM Modulator long prefix/1 -> data_out/1

== system tx2/Subsystem8/OFDM_process1/OFDM_process1_bf3/ctrl_gen ==
  data_in : Inport
      settings: SignalType=complex
  valid_in : Inport  Port=2
  Delay : Delay  DelayLength=1  InitialCondition=0
  Delay1 : Delay  DelayLength=1  InitialCondition=0
  Delay2 : Delay  DelayLength=1  InitialCondition=0
  Detect Fall Nonpositive : hdlsllib/Logic and Bit Operations/Detect Fall Nonpositive  vinit=0  OutDataTypeStr=boolean
      settings: SourceProductBaseCode=SL
  Detect Rise Positive : hdlsllib/Logic and Bit Operations/Detect Rise Positive  vinit=0  OutDataTypeStr=boolean
      settings: SourceProductBaseCode=SL
  Sample Control Bus Creator : whdlutilities/Sample Control Bus Creator
      settings: SourceProductBaseCode=LH
  data_out : Outport
  ctrl_out : Outport  Port=2
  wires:
  Detect Fall Nonpositive/1 -> Sample Control Bus Creator/2
  Detect Rise Positive/1 -> Sample Control Bus Creator/1
  valid_in/1 -> Delay/1, Detect Fall Nonpositive/1, Delay1/1
  Sample Control Bus Creator/1 -> ctrl_out/1
  Delay/1 -> Sample Control Bus Creator/3
  Delay1/1 -> Detect Rise Positive/1
  data_in/1 -> Delay2/1
  Delay2/1 -> data_out/1
